simulink model "Systolic_4x4"  (R2021a)
settings: Solver=VariableStepAuto  StartTime=0.0  StopTime=32  RelTol=1e-3
libraries: hdlBasic x195, xbsIndex_r4 x1
(part 1 of 2)
settings Model: Creator=ckk5  LastModifiedBy=ckk5

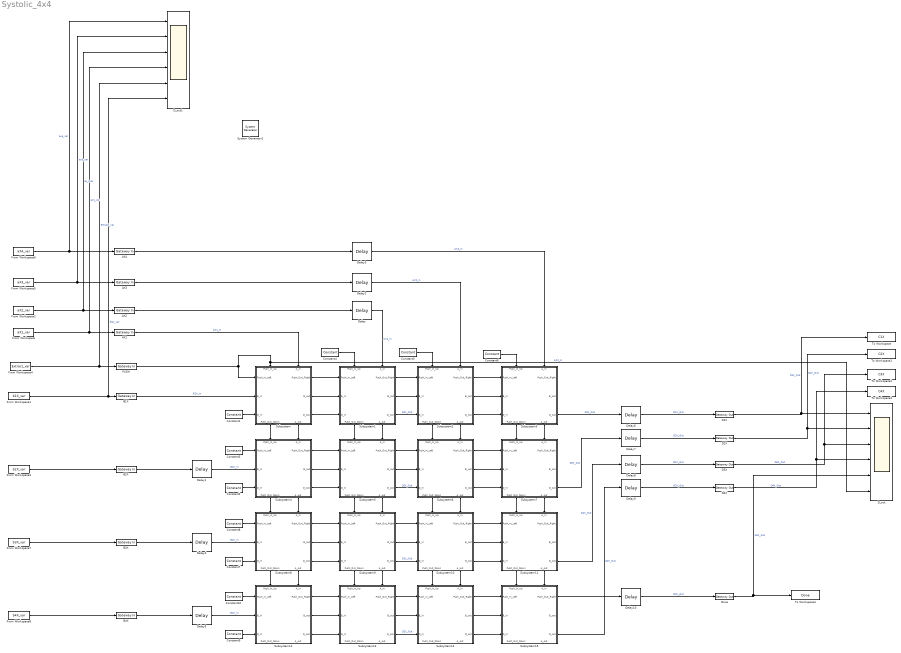
== system Systolic_4x4 ==
  " System Generator1" : xbsIndex_r4/ System Generator  Tag=genX  xilinxfamily=zynq  part=xc7z020  speed=-1  package=clg484  synthesis_tool=Vivado  clock_wrapper=Clock Enables  directory=C:/ELEC522/Cameron/systolic_array_shit  proj_type=Vivado  Synth_file=Vivado Synthesis Defaults  Impl_file=Vivado Implementation Defaults  testbench=off  simulink_period=1  sysclk_period=10  dcm_input_clock_period=10  incr_netlist=off  trim_vbits=Everywhere in SubSystem  dbl_ovrd=According to Block Masks  core_generation=According to Block Masks  run_coregen=off  deprecated_control=off  eval_field=0  block_type=sysgen
  AX{1..4} (4 alike) : hdlBasic/Gateway In  gui_display_data_type=Fixed-point  arith_type=Signed (2's comp)  n_bits=16  bin_pt=0  preci_type=Single  exp_width=8  frac_width=24  rows=1  columns=1  quantization="Round  (unbiased: +/- Inf)"  overflow=Saturate  period=1  UseAsADC=off  ADCChannel='1'  interface=None  automatic_assignment=on  address_offset=hex2dec('00')  intf_name=''  intf_description=''  default_value=0  timing_constraint=None  locs_specified=off  LOCs={}  io_standard={}  inherit_from_input=off  hdl_port=on  XmcBlockStatus=1  maskContainerNames=group4  block_type=gatewayin  block_config=sysgen:gateway_in_config  block_width_w=590  block_height_w=620  block_width=640  block_height=850
  B1X : hdlBasic/Gateway In  gui_display_data_type=Fixed-point  arith_type=Signed (2's comp)  n_bits=16  bin_pt=0  preci_type=Single  exp_width=8  frac_width=24  rows=1  columns=1  quantization="Round  (unbiased: +/- Inf)"  overflow=Saturate  period=1  UseAsADC=off  ADCChannel='1'  interface=None  automatic_assignment=on  address_offset=hex2dec('00')  intf_name=''  intf_description=''  default_value=0  timing_constraint=None  locs_specified=off  LOCs={}  io_standard={}  inherit_from_input=off  hdl_port=on  XmcBlockStatus=1  maskContainerNames=group4  block_type=gatewayin  block_config=sysgen:gateway_in_config  block_width_w=590  block_height_w=620  block_width=640  block_height=850
  B2X : hdlBasic/Gateway In  gui_display_data_type=Fixed-point  arith_type=Signed (2's comp)  n_bits=16  bin_pt=0  preci_type=Single  exp_width=8  frac_width=24  rows=1  columns=1  quantization="Round  (unbiased: +/- Inf)"  overflow=Saturate  period=1  UseAsADC=off  ADCChannel='1'  interface=None  automatic_assignment=on  address_offset=hex2dec('00')  intf_name=''  intf_description=''  default_value=0  timing_constraint=None  locs_specified=off  LOCs={}  io_standard={}  inherit_from_input=off  hdl_port=on  XmcBlockStatus=1  maskContainerNames=group4  block_type=gatewayin  block_config=sysgen:gateway_in_config  block_width_w=590  block_height_w=620  block_width=640  block_height=850
  B3X : hdlBasic/Gateway In  gui_display_data_type=Fixed-point  arith_type=Signed (2's comp)  n_bits=16  bin_pt=0  preci_type=Single  exp_width=8  frac_width=24  rows=1  columns=1  quantization="Round  (unbiased: +/- Inf)"  overflow=Saturate  period=1  UseAsADC=off  ADCChannel='1'  interface=None  automatic_assignment=on  address_offset=hex2dec('00')  intf_name=''  intf_description=''  default_value=0  timing_constraint=None  locs_specified=off  LOCs={}  io_standard={}  inherit_from_input=off  hdl_port=on  XmcBlockStatus=1  maskContainerNames=group4  block_type=gatewayin  block_config=sysgen:gateway_in_config  block_width_w=590  block_height_w=620  block_width=640  block_height=850
  B4X : hdlBasic/Gateway In  gui_display_data_type=Fixed-point  arith_type=Signed (2's comp)  n_bits=16  bin_pt=0  preci_type=Single  exp_width=8  frac_width=24  rows=1  columns=1  quantization="Round  (unbiased: +/- Inf)"  overflow=Saturate  period=1  UseAsADC=off  ADCChannel='1'  interface=None  automatic_assignment=on  address_offset=hex2dec('00')  intf_name=''  intf_description=''  default_value=0  timing_constraint=None  locs_specified=off  LOCs={}  io_standard={}  inherit_from_input=off  hdl_port=on  XmcBlockStatus=1  maskContainerNames=group4  block_type=gatewayin  block_config=sysgen:gateway_in_config  block_width_w=590  block_height_w=620  block_width=640  block_height=850
  Constant{1..2,7,9} (4 alike) : hdlBasic/Constant  const=0  gui_display_data_type=Fixed-point  arith_type=Signed (2's comp)  n_bits=16  bin_pt=0  preci_type=Single  exp_width=8  frac_width=24  explicit_period=off  period=1  XmcBlockStatus=1  maskContainerNames=tabcontainer1  block_type=constant  block_config=sysgen:Constant_config
  Constant{3..6,8,10} (6 alike) : hdlBasic/Constant  const=0  gui_display_data_type=Boolean  arith_type=Boolean  n_bits=16  bin_pt=0  preci_type=Single  exp_width=8  frac_width=24  explicit_period=off  period=1  XmcBlockStatus=1  maskContainerNames=tabcontainer1  block_type=constant  block_config=sysgen:Constant_config
  D1X : hdlBasic/Gateway Out  inherit_from_input=off  hdl_port=on  rows=1  columns=1  UseAsDAC=off  DACChannel='1'  interface=None  automatic_assignment=on  address_offset=hex2dec('00')  intf_name=''  intf_description=''  timing_constraint=None  locs_specified=off  LOCs={}  io_standard={}  XmcBlockStatus=1  maskContainerNames=group4  block_type=gatewayout  block_config=sysgen:gateway_out_config  block_width_w=590  block_height_w=620  block_width=620  block_height=750
  D2X : hdlBasic/Gateway Out  inherit_from_input=off  hdl_port=on  rows=1  columns=1  UseAsDAC=off  DACChannel='1'  interface=None  automatic_assignment=on  address_offset=hex2dec('00')  intf_name=''  intf_description=''  timing_constraint=None  locs_specified=off  LOCs={}  io_standard={}  XmcBlockStatus=1  maskContainerNames=group4  block_type=gatewayout  block_config=sysgen:gateway_out_config  block_width_w=590  block_height_w=620  block_width=620  block_height=750
  D3X : hdlBasic/Gateway Out  inherit_from_input=off  hdl_port=on  rows=1  columns=1  UseAsDAC=off  DACChannel='1'  interface=None  automatic_assignment=on  address_offset=hex2dec('00')  intf_name=''  intf_description=''  timing_constraint=None  locs_specified=off  LOCs={}  io_standard={}  XmcBlockStatus=1  maskContainerNames=group4  block_type=gatewayout  block_config=sysgen:gateway_out_config  block_width_w=590  block_height_w=620  block_width=620  block_height=750
  D4X : hdlBasic/Gateway Out  inherit_from_input=off  hdl_port=on  rows=1  columns=1  UseAsDAC=off  DACChannel='1'  interface=None  automatic_assignment=on  address_offset=hex2dec('00')  intf_name=''  intf_description=''  timing_constraint=None  locs_specified=off  LOCs={}  io_standard={}  XmcBlockStatus=1  maskContainerNames=group4  block_type=gatewayout  block_config=sysgen:gateway_out_config  block_width_w=590  block_height_w=620  block_width=620  block_height=750
  D_out : Scope  NumInputPorts=6
  D_out1 : Scope  NumInputPorts=6
  Delay{,1,9..10} (4 alike) : hdlBasic/Delay  rst=off  en=off  latency=1  reg_retiming=off  XmcBlockStatus=1  maskContainerNames=group1  block_type=delay  block_config=sysgen:Delay_config
  Delay2 : hdlBasic/Delay  rst=off  en=off  latency=2  reg_retiming=off  XmcBlockStatus=1  maskContainerNames=group1  block_type=delay  block_config=sysgen:Delay_config
  Delay3 : hdlBasic/Delay  rst=off  en=off  latency=3  reg_retiming=off  XmcBlockStatus=1  maskContainerNames=group1  block_type=delay  block_config=sysgen:Delay_config
  Delay4 : hdlBasic/Delay  rst=off  en=off  latency=2  reg_retiming=off  XmcBlockStatus=1  maskContainerNames=group1  block_type=delay  block_config=sysgen:Delay_config
  Delay5 : hdlBasic/Delay  rst=off  en=off  latency=3  reg_retiming=off  XmcBlockStatus=1  maskContainerNames=group1  block_type=delay  block_config=sysgen:Delay_config
  Delay6 : hdlBasic/Delay  rst=off  en=off  latency=4  reg_retiming=off  XmcBlockStatus=1  maskContainerNames=group1  block_type=delay  block_config=sysgen:Delay_config
  Delay7 : hdlBasic/Delay  rst=off  en=off  latency=3  reg_retiming=off  XmcBlockStatus=1  maskContainerNames=group1  block_type=delay  block_config=sysgen:Delay_config
  Delay8 : hdlBasic/Delay  rst=off  en=off  latency=2  reg_retiming=off  XmcBlockStatus=1  maskContainerNames=group1  block_type=delay  block_config=sysgen:Delay_config
  Done : hdlBasic/Gateway Out  inherit_from_input=off  hdl_port=on  rows=1  columns=1  UseAsDAC=off  DACChannel='1'  interface=None  automatic_assignment=on  address_offset=hex2dec('00')  intf_name=''  intf_description=''  timing_constraint=None  locs_specified=off  LOCs={}  io_standard={}  XmcBlockStatus=1  maskContainerNames=group4  block_type=gatewayout  block_config=sysgen:gateway_out_config  block_width_w=590  block_height_w=620  block_width=620  block_height=750
  From Workspace : FromWorkspace  VariableName=aX1_var  Interpolate=off  OutputAfterFinalValue=Setting to zero
  From Workspace1 : FromWorkspace  VariableName=b1X_var  Interpolate=off  OutputAfterFinalValue=Setting to zero
  From Workspace2 : FromWorkspace  VariableName=aX2_var  Interpolate=off  OutputAfterFinalValue=Setting to zero
  From Workspace3 : FromWorkspace  VariableName=b2X_var  Interpolate=off  OutputAfterFinalValue=Setting to zero
  From Workspace4 : FromWorkspace  VariableName=Extract_var  Interpolate=off  OutputAfterFinalValue=Setting to zero
  From Workspace5 : FromWorkspace  VariableName=aX3_var  Interpolate=off  OutputAfterFinalValue=Setting to zero
  From Workspace6 : FromWorkspace  VariableName=aX4_var  Interpolate=off  OutputAfterFinalValue=Setting to zero
  From Workspace7 : FromWorkspace  VariableName=b3X_var  Interpolate=off  OutputAfterFinalValue=Setting to zero
  From Workspace8 : FromWorkspace  VariableName=b4X_var  Interpolate=off  OutputAfterFinalValue=Setting to zero
  PUSH : hdlBasic/Gateway In  gui_display_data_type=Boolean  arith_type=Boolean  n_bits=1  bin_pt=0  preci_type=Single  exp_width=8  frac_width=24  rows=1  columns=1  quantization="Round  (unbiased: +/- Inf)"  overflow=Saturate  period=1  UseAsADC=off  ADCChannel='1'  interface=None  automatic_assignment=on  address_offset=hex2dec('00')  intf_name=''  intf_description=''  default_value=0  timing_constraint=None  locs_specified=off  LOCs={}  io_standard={}  inherit_from_input=off  hdl_port=on  XmcBlockStatus=1  maskContainerNames=group4  block_type=gatewayin  block_config=sysgen:gateway_in_config  block_width_w=590  block_height_w=620  block_width=640  block_height=850
  Subsystem : Subsystem
      settings: PortSchema="{\"entries\":[{\"content\":{\"sides\":[{\"content\":{\"connectorIds\":[\"In1\",\"In2\",\"In3\"]},\"type\":\"ConnectorPlacement.EquallySpacedRectSide\",\"uuid\":\"8ff87642-4ab4-4993-8c2d-3e2a0b442edb\"},{\"content\":{\"connectorIds\":[\"Out1\",\"Out2\",\"Out3\"],\"side\":\"RIGHT\"},\"type\":\"ConnectorPlacement.EquallySpacedRectSide\",\"uuid\":\"3e5e616f-4833-4873-80b3-d7c022d50595\"},{\"content\":{\"connectorIds\":[\"In4\",\"In5\"],\"side\":\"TOP\"},\"type\":\"ConnectorPlacement.EquallySpacedRectSide\",\"uuid\":\"e9723aa0-a983-4533-a9ef-daafc8525bc8\"},{\"content\":{\"connectorIds\":[\"Out4\",\"Out5\"],\"side\":\"BOTTOM\"},\"type\":\"ConnectorPlacement.EquallySpacedRectSide\",\"uuid\":\"893be137-9383-4d88-a8a8-bff1bf557b52\"}]},\"type\":\"ConnectorPlacement.EquallySpacedConnector\",\"uuid\":\"84d6313b-76ca-421f-b981-b36aad77f192\"}],\"packageUris\":[\"http://schema.mathworks.com/mf0/Connector/R2020b\"],\"version\":\"1.0\"}"
  Subsystem1 : Subsystem
      settings: PortSchema="{\"entries\":[{\"content\":{\"sides\":[{\"content\":{\"connectorIds\":[\"In1\",\"In2\",\"In3\"]},\"type\":\"ConnectorPlacement.EquallySpacedRectSide\",\"uuid\":\"8ff87642-4ab4-4993-8c2d-3e2a0b442edb\"},{\"content\":{\"connectorIds\":[\"Out1\",\"Out2\",\"Out3\"],\"side\":\"RIGHT\"},\"type\":\"ConnectorPlacement.EquallySpacedRectSide\",\"uuid\":\"3e5e616f-4833-4873-80b3-d7c022d50595\"},{\"content\":{\"connectorIds\":[\"In4\",\"In5\"],\"side\":\"TOP\"},\"type\":\"ConnectorPlacement.EquallySpacedRectSide\",\"uuid\":\"e9723aa0-a983-4533-a9ef-daafc8525bc8\"},{\"content\":{\"connectorIds\":[\"Out4\",\"Out5\"],\"side\":\"BOTTOM\"},\"type\":\"ConnectorPlacement.EquallySpacedRectSide\",\"uuid\":\"893be137-9383-4d88-a8a8-bff1bf557b52\"}]},\"type\":\"ConnectorPlacement.EquallySpacedConnector\",\"uuid\":\"84d6313b-76ca-421f-b981-b36aad77f192\"}],\"packageUris\":[\"http://schema.mathworks.com/mf0/Connector/R2020b\"],\"version\":\"1.0\"}"
  Subsystem10 : Subsystem
      settings: PortSchema="{\"entries\":[{\"content\":{\"sides\":[{\"content\":{\"connectorIds\":[\"In1\",\"In2\",\"In3\"]},\"type\":\"ConnectorPlacement.EquallySpacedRectSide\",\"uuid\":\"8ff87642-4ab4-4993-8c2d-3e2a0b442edb\"},{\"content\":{\"connectorIds\":[\"Out1\",\"Out2\",\"Out3\"],\"side\":\"RIGHT\"},\"type\":\"ConnectorPlacement.EquallySpacedRectSide\",\"uuid\":\"3e5e616f-4833-4873-80b3-d7c022d50595\"},{\"content\":{\"connectorIds\":[\"In4\",\"In5\"],\"side\":\"TOP\"},\"type\":\"ConnectorPlacement.EquallySpacedRectSide\",\"uuid\":\"e9723aa0-a983-4533-a9ef-daafc8525bc8\"},{\"content\":{\"connectorIds\":[\"Out4\",\"Out5\"],\"side\":\"BOTTOM\"},\"type\":\"ConnectorPlacement.EquallySpacedRectSide\",\"uuid\":\"893be137-9383-4d88-a8a8-bff1bf557b52\"}]},\"type\":\"ConnectorPlacement.EquallySpacedConnector\",\"uuid\":\"84d6313b-76ca-421f-b981-b36aad77f192\"}],\"packageUris\":[\"http://schema.mathworks.com/mf0/Connector/R2020b\"],\"version\":\"1.0\"}"
  Subsystem11 : Subsystem
      settings: PortSchema="{\"entries\":[{\"content\":{\"sides\":[{\"content\":{\"connectorIds\":[\"In1\",\"In2\",\"In3\"]},\"type\":\"ConnectorPlacement.EquallySpacedRectSide\",\"uuid\":\"8ff87642-4ab4-4993-8c2d-3e2a0b442edb\"},{\"content\":{\"connectorIds\":[\"Out1\",\"Out2\",\"Out3\"],\"side\":\"RIGHT\"},\"type\":\"ConnectorPlacement.EquallySpacedRectSide\",\"uuid\":\"3e5e616f-4833-4873-80b3-d7c022d50595\"},{\"content\":{\"connectorIds\":[\"In4\",\"In5\"],\"side\":\"TOP\"},\"type\":\"ConnectorPlacement.EquallySpacedRectSide\",\"uuid\":\"e9723aa0-a983-4533-a9ef-daafc8525bc8\"},{\"content\":{\"connectorIds\":[\"Out4\",\"Out5\"],\"side\":\"BOTTOM\"},\"type\":\"ConnectorPlacement.EquallySpacedRectSide\",\"uuid\":\"893be137-9383-4d88-a8a8-bff1bf557b52\"}]},\"type\":\"ConnectorPlacement.EquallySpacedConnector\",\"uuid\":\"84d6313b-76ca-421f-b981-b36aad77f192\"}],\"packageUris\":[\"http://schema.mathworks.com/mf0/Connector/R2020b\"],\"version\":\"1.0\"}"
  Subsystem12 : Subsystem
      settings: PortSchema="{\"entries\":[{\"content\":{\"sides\":[{\"content\":{\"connectorIds\":[\"In1\",\"In2\",\"In3\"]},\"type\":\"ConnectorPlacement.EquallySpacedRectSide\",\"uuid\":\"8ff87642-4ab4-4993-8c2d-3e2a0b442edb\"},{\"content\":{\"connectorIds\":[\"Out1\",\"Out2\",\"Out3\"],\"side\":\"RIGHT\"},\"type\":\"ConnectorPlacement.EquallySpacedRectSide\",\"uuid\":\"3e5e616f-4833-4873-80b3-d7c022d50595\"},{\"content\":{\"connectorIds\":[\"In4\",\"In5\"],\"side\":\"TOP\"},\"type\":\"ConnectorPlacement.EquallySpacedRectSide\",\"uuid\":\"e9723aa0-a983-4533-a9ef-daafc8525bc8\"},{\"content\":{\"connectorIds\":[\"Out4\",\"Out5\"],\"side\":\"BOTTOM\"},\"type\":\"ConnectorPlacement.EquallySpacedRectSide\",\"uuid\":\"893be137-9383-4d88-a8a8-bff1bf557b52\"}]},\"type\":\"ConnectorPlacement.EquallySpacedConnector\",\"uuid\":\"84d6313b-76ca-421f-b981-b36aad77f192\"}],\"packageUris\":[\"http://schema.mathworks.com/mf0/Connector/R2020b\"],\"version\":\"1.0\"}"
  Subsystem13 : Subsystem
      settings: PortSchema="{\"entries\":[{\"content\":{\"sides\":[{\"content\":{\"connectorIds\":[\"In1\",\"In2\",\"In3\"]},\"type\":\"ConnectorPlacement.EquallySpacedRectSide\",\"uuid\":\"8ff87642-4ab4-4993-8c2d-3e2a0b442edb\"},{\"content\":{\"connectorIds\":[\"Out1\",\"Out2\",\"Out3\"],\"side\":\"RIGHT\"},\"type\":\"ConnectorPlacement.EquallySpacedRectSide\",\"uuid\":\"3e5e616f-4833-4873-80b3-d7c022d50595\"},{\"content\":{\"connectorIds\":[\"In4\",\"In5\"],\"side\":\"TOP\"},\"type\":\"ConnectorPlacement.EquallySpacedRectSide\",\"uuid\":\"e9723aa0-a983-4533-a9ef-daafc8525bc8\"},{\"content\":{\"connectorIds\":[\"Out4\",\"Out5\"],\"side\":\"BOTTOM\"},\"type\":\"ConnectorPlacement.EquallySpacedRectSide\",\"uuid\":\"893be137-9383-4d88-a8a8-bff1bf557b52\"}]},\"type\":\"ConnectorPlacement.EquallySpacedConnector\",\"uuid\":\"84d6313b-76ca-421f-b981-b36aad77f192\"}],\"packageUris\":[\"http://schema.mathworks.com/mf0/Connector/R2020b\"],\"version\":\"1.0\"}"
  Subsystem14 : Subsystem
      settings: PortSchema="{\"entries\":[{\"content\":{\"sides\":[{\"content\":{\"connectorIds\":[\"In1\",\"In2\",\"In3\"]},\"type\":\"ConnectorPlacement.EquallySpacedRectSide\",\"uuid\":\"8ff87642-4ab4-4993-8c2d-3e2a0b442edb\"},{\"content\":{\"connectorIds\":[\"Out1\",\"Out2\",\"Out3\"],\"side\":\"RIGHT\"},\"type\":\"ConnectorPlacement.EquallySpacedRectSide\",\"uuid\":\"3e5e616f-4833-4873-80b3-d7c022d50595\"},{\"content\":{\"connectorIds\":[\"In4\",\"In5\"],\"side\":\"TOP\"},\"type\":\"ConnectorPlacement.EquallySpacedRectSide\",\"uuid\":\"e9723aa0-a983-4533-a9ef-daafc8525bc8\"},{\"content\":{\"connectorIds\":[\"Out4\",\"Out5\"],\"side\":\"BOTTOM\"},\"type\":\"ConnectorPlacement.EquallySpacedRectSide\",\"uuid\":\"893be137-9383-4d88-a8a8-bff1bf557b52\"}]},\"type\":\"ConnectorPlacement.EquallySpacedConnector\",\"uuid\":\"84d6313b-76ca-421f-b981-b36aad77f192\"}],\"packageUris\":[\"http://schema.mathworks.com/mf0/Connector/R2020b\"],\"version\":\"1.0\"}"
  Subsystem15 : Subsystem
      settings: PortSchema="{\"entries\":[{\"content\":{\"sides\":[{\"content\":{\"connectorIds\":[\"In1\",\"In2\",\"In3\"]},\"type\":\"ConnectorPlacement.EquallySpacedRectSide\",\"uuid\":\"8ff87642-4ab4-4993-8c2d-3e2a0b442edb\"},{\"content\":{\"connectorIds\":[\"Out1\",\"Out2\",\"Out3\"],\"side\":\"RIGHT\"},\"type\":\"ConnectorPlacement.EquallySpacedRectSide\",\"uuid\":\"3e5e616f-4833-4873-80b3-d7c022d50595\"},{\"content\":{\"connectorIds\":[\"In4\",\"In5\"],\"side\":\"TOP\"},\"type\":\"ConnectorPlacement.EquallySpacedRectSide\",\"uuid\":\"e9723aa0-a983-4533-a9ef-daafc8525bc8\"},{\"content\":{\"connectorIds\":[\"Out4\",\"Out5\"],\"side\":\"BOTTOM\"},\"type\":\"ConnectorPlacement.EquallySpacedRectSide\",\"uuid\":\"893be137-9383-4d88-a8a8-bff1bf557b52\"}]},\"type\":\"ConnectorPlacement.EquallySpacedConnector\",\"uuid\":\"84d6313b-76ca-421f-b981-b36aad77f192\"}],\"packageUris\":[\"http://schema.mathworks.com/mf0/Connector/R2020b\"],\"version\":\"1.0\"}"
  Subsystem2 : Subsystem
      settings: PortSchema="{\"entries\":[{\"content\":{\"sides\":[{\"content\":{\"connectorIds\":[\"In1\",\"In2\",\"In3\"]},\"type\":\"ConnectorPlacement.EquallySpacedRectSide\",\"uuid\":\"8ff87642-4ab4-4993-8c2d-3e2a0b442edb\"},{\"content\":{\"connectorIds\":[\"Out1\",\"Out2\",\"Out3\"],\"side\":\"RIGHT\"},\"type\":\"ConnectorPlacement.EquallySpacedRectSide\",\"uuid\":\"3e5e616f-4833-4873-80b3-d7c022d50595\"},{\"content\":{\"connectorIds\":[\"In4\",\"In5\"],\"side\":\"TOP\"},\"type\":\"ConnectorPlacement.EquallySpacedRectSide\",\"uuid\":\"e9723aa0-a983-4533-a9ef-daafc8525bc8\"},{\"content\":{\"connectorIds\":[\"Out4\",\"Out5\"],\"side\":\"BOTTOM\"},\"type\":\"ConnectorPlacement.EquallySpacedRectSide\",\"uuid\":\"893be137-9383-4d88-a8a8-bff1bf557b52\"}]},\"type\":\"ConnectorPlacement.EquallySpacedConnector\",\"uuid\":\"84d6313b-76ca-421f-b981-b36aad77f192\"}],\"packageUris\":[\"http://schema.mathworks.com/mf0/Connector/R2020b\"],\"version\":\"1.0\"}"
  Subsystem3 : Subsystem
      settings: PortSchema="{\"entries\":[{\"content\":{\"sides\":[{\"content\":{\"connectorIds\":[\"In1\",\"In2\",\"In3\"]},\"type\":\"ConnectorPlacement.EquallySpacedRectSide\",\"uuid\":\"8ff87642-4ab4-4993-8c2d-3e2a0b442edb\"},{\"content\":{\"connectorIds\":[\"Out1\",\"Out2\",\"Out3\"],\"side\":\"RIGHT\"},\"type\":\"ConnectorPlacement.EquallySpacedRectSide\",\"uuid\":\"3e5e616f-4833-4873-80b3-d7c022d50595\"},{\"content\":{\"connectorIds\":[\"In4\",\"In5\"],\"side\":\"TOP\"},\"type\":\"ConnectorPlacement.EquallySpacedRectSide\",\"uuid\":\"e9723aa0-a983-4533-a9ef-daafc8525bc8\"},{\"content\":{\"connectorIds\":[\"Out4\",\"Out5\"],\"side\":\"BOTTOM\"},\"type\":\"ConnectorPlacement.EquallySpacedRectSide\",\"uuid\":\"893be137-9383-4d88-a8a8-bff1bf557b52\"}]},\"type\":\"ConnectorPlacement.EquallySpacedConnector\",\"uuid\":\"84d6313b-76ca-421f-b981-b36aad77f192\"}],\"packageUris\":[\"http://schema.mathworks.com/mf0/Connector/R2020b\"],\"version\":\"1.0\"}"
  Subsystem4 : Subsystem
      settings: PortSchema="{\"entries\":[{\"content\":{\"sides\":[{\"content\":{\"connectorIds\":[\"In1\",\"In2\",\"In3\"]},\"type\":\"ConnectorPlacement.EquallySpacedRectSide\",\"uuid\":\"8ff87642-4ab4-4993-8c2d-3e2a0b442edb\"},{\"content\":{\"connectorIds\":[\"Out1\",\"Out2\",\"Out3\"],\"side\":\"RIGHT\"},\"type\":\"ConnectorPlacement.EquallySpacedRectSide\",\"uuid\":\"3e5e616f-4833-4873-80b3-d7c022d50595\"},{\"content\":{\"connectorIds\":[\"In4\",\"In5\"],\"side\":\"TOP\"},\"type\":\"ConnectorPlacement.EquallySpacedRectSide\",\"uuid\":\"e9723aa0-a983-4533-a9ef-daafc8525bc8\"},{\"content\":{\"connectorIds\":[\"Out4\",\"Out5\"],\"side\":\"BOTTOM\"},\"type\":\"ConnectorPlacement.EquallySpacedRectSide\",\"uuid\":\"893be137-9383-4d88-a8a8-bff1bf557b52\"}]},\"type\":\"ConnectorPlacement.EquallySpacedConnector\",\"uuid\":\"84d6313b-76ca-421f-b981-b36aad77f192\"}],\"packageUris\":[\"http://schema.mathworks.com/mf0/Connector/R2020b\"],\"version\":\"1.0\"}"
  Subsystem5 : Subsystem
      settings: PortSchema="{\"entries\":[{\"content\":{\"sides\":[{\"content\":{\"connectorIds\":[\"In1\",\"In2\",\"In3\"]},\"type\":\"ConnectorPlacement.EquallySpacedRectSide\",\"uuid\":\"8ff87642-4ab4-4993-8c2d-3e2a0b442edb\"},{\"content\":{\"connectorIds\":[\"Out1\",\"Out2\",\"Out3\"],\"side\":\"RIGHT\"},\"type\":\"ConnectorPlacement.EquallySpacedRectSide\",\"uuid\":\"3e5e616f-4833-4873-80b3-d7c022d50595\"},{\"content\":{\"connectorIds\":[\"In4\",\"In5\"],\"side\":\"TOP\"},\"type\":\"ConnectorPlacement.EquallySpacedRectSide\",\"uuid\":\"e9723aa0-a983-4533-a9ef-daafc8525bc8\"},{\"content\":{\"connectorIds\":[\"Out4\",\"Out5\"],\"side\":\"BOTTOM\"},\"type\":\"ConnectorPlacement.EquallySpacedRectSide\",\"uuid\":\"893be137-9383-4d88-a8a8-bff1bf557b52\"}]},\"type\":\"ConnectorPlacement.EquallySpacedConnector\",\"uuid\":\"84d6313b-76ca-421f-b981-b36aad77f192\"}],\"packageUris\":[\"http://schema.mathworks.com/mf0/Connector/R2020b\"],\"version\":\"1.0\"}"
  Subsystem6 : Subsystem
      settings: PortSchema="{\"entries\":[{\"content\":{\"sides\":[{\"content\":{\"connectorIds\":[\"In1\",\"In2\",\"In3\"]},\"type\":\"ConnectorPlacement.EquallySpacedRectSide\",\"uuid\":\"8ff87642-4ab4-4993-8c2d-3e2a0b442edb\"},{\"content\":{\"connectorIds\":[\"Out1\",\"Out2\",\"Out3\"],\"side\":\"RIGHT\"},\"type\":\"ConnectorPlacement.EquallySpacedRectSide\",\"uuid\":\"3e5e616f-4833-4873-80b3-d7c022d50595\"},{\"content\":{\"connectorIds\":[\"In4\",\"In5\"],\"side\":\"TOP\"},\"type\":\"ConnectorPlacement.EquallySpacedRectSide\",\"uuid\":\"e9723aa0-a983-4533-a9ef-daafc8525bc8\"},{\"content\":{\"connectorIds\":[\"Out4\",\"Out5\"],\"side\":\"BOTTOM\"},\"type\":\"ConnectorPlacement.EquallySpacedRectSide\",\"uuid\":\"893be137-9383-4d88-a8a8-bff1bf557b52\"}]},\"type\":\"ConnectorPlacement.EquallySpacedConnector\",\"uuid\":\"84d6313b-76ca-421f-b981-b36aad77f192\"}],\"packageUris\":[\"http://schema.mathworks.com/mf0/Connector/R2020b\"],\"version\":\"1.0\"}"
  Subsystem7 : Subsystem
      settings: PortSchema="{\"entries\":[{\"content\":{\"sides\":[{\"content\":{\"connectorIds\":[\"In1\",\"In2\",\"In3\"]},\"type\":\"ConnectorPlacement.EquallySpacedRectSide\",\"uuid\":\"8ff87642-4ab4-4993-8c2d-3e2a0b442edb\"},{\"content\":{\"connectorIds\":[\"Out1\",\"Out2\",\"Out3\"],\"side\":\"RIGHT\"},\"type\":\"ConnectorPlacement.EquallySpacedRectSide\",\"uuid\":\"3e5e616f-4833-4873-80b3-d7c022d50595\"},{\"content\":{\"connectorIds\":[\"In4\",\"In5\"],\"side\":\"TOP\"},\"type\":\"ConnectorPlacement.EquallySpacedRectSide\",\"uuid\":\"e9723aa0-a983-4533-a9ef-daafc8525bc8\"},{\"content\":{\"connectorIds\":[\"Out4\",\"Out5\"],\"side\":\"BOTTOM\"},\"type\":\"ConnectorPlacement.EquallySpacedRectSide\",\"uuid\":\"893be137-9383-4d88-a8a8-bff1bf557b52\"}]},\"type\":\"ConnectorPlacement.EquallySpacedConnector\",\"uuid\":\"84d6313b-76ca-421f-b981-b36aad77f192\"}],\"packageUris\":[\"http://schema.mathworks.com/mf0/Connector/R2020b\"],\"version\":\"1.0\"}"
  Subsystem8 : Subsystem
      settings: PortSchema="{\"entries\":[{\"content\":{\"sides\":[{\"content\":{\"connectorIds\":[\"In1\",\"In2\",\"In3\"]},\"type\":\"ConnectorPlacement.EquallySpacedRectSide\",\"uuid\":\"8ff87642-4ab4-4993-8c2d-3e2a0b442edb\"},{\"content\":{\"connectorIds\":[\"Out1\",\"Out2\",\"Out3\"],\"side\":\"RIGHT\"},\"type\":\"ConnectorPlacement.EquallySpacedRectSide\",\"uuid\":\"3e5e616f-4833-4873-80b3-d7c022d50595\"},{\"content\":{\"connectorIds\":[\"In4\",\"In5\"],\"side\":\"TOP\"},\"type\":\"ConnectorPlacement.EquallySpacedRectSide\",\"uuid\":\"e9723aa0-a983-4533-a9ef-daafc8525bc8\"},{\"content\":{\"connectorIds\":[\"Out4\",\"Out5\"],\"side\":\"BOTTOM\"},\"type\":\"ConnectorPlacement.EquallySpacedRectSide\",\"uuid\":\"893be137-9383-4d88-a8a8-bff1bf557b52\"}]},\"type\":\"ConnectorPlacement.EquallySpacedConnector\",\"uuid\":\"84d6313b-76ca-421f-b981-b36aad77f192\"}],\"packageUris\":[\"http://schema.mathworks.com/mf0/Connector/R2020b\"],\"version\":\"1.0\"}"
  Subsystem9 : Subsystem
      settings: PortSchema="{\"entries\":[{\"content\":{\"sides\":[{\"content\":{\"connectorIds\":[\"In1\",\"In2\",\"In3\"]},\"type\":\"ConnectorPlacement.EquallySpacedRectSide\",\"uuid\":\"8ff87642-4ab4-4993-8c2d-3e2a0b442edb\"},{\"content\":{\"connectorIds\":[\"Out1\",\"Out2\",\"Out3\"],\"side\":\"RIGHT\"},\"type\":\"ConnectorPlacement.EquallySpacedRectSide\",\"uuid\":\"3e5e616f-4833-4873-80b3-d7c022d50595\"},{\"content\":{\"connectorIds\":[\"In4\",\"In5\"],\"side\":\"TOP\"},\"type\":\"ConnectorPlacement.EquallySpacedRectSide\",\"uuid\":\"e9723aa0-a983-4533-a9ef-daafc8525bc8\"},{\"content\":{\"connectorIds\":[\"Out4\",\"Out5\"],\"side\":\"BOTTOM\"},\"type\":\"ConnectorPlacement.EquallySpacedRectSide\",\"uuid\":\"893be137-9383-4d88-a8a8-bff1bf557b52\"}]},\"type\":\"ConnectorPlacement.EquallySpacedConnector\",\"uuid\":\"84d6313b-76ca-421f-b981-b36aad77f192\"}],\"packageUris\":[\"http://schema.mathworks.com/mf0/Connector/R2020b\"],\"version\":\"1.0\"}"
  To Workspace : ToWorkspace  VariableName=C1X  SaveFormat=Timeseries  SampleTime=-1
  To Workspace1 : ToWorkspace  VariableName=C2X  SaveFormat=Timeseries  SampleTime=-1
  To Workspace2 : ToWorkspace  VariableName=C3X  SaveFormat=Timeseries  SampleTime=-1
  To Workspace3 : ToWorkspace  VariableName=C4X  SaveFormat=Timeseries  SampleTime=-1
  To Workspace4 : ToWorkspace  VariableName=Done  SaveFormat=Timeseries  SampleTime=-1
  wires:
  From Workspace/1 -> D_out1/4, AX1/1  "ax1_var"
  AX1/1 -> Subsystem/5(A_in)  "AX1_In"
  From Workspace1/1 -> D_out1/6, B1X/1  "B1x_var"
  B1X/1 -> Subsystem/2(B_in)  "B1X_In"
  Subsystem1/5(A_out) -> Subsystem5/5(A_in)
  Subsystem1/4(Push_Out_Down) -> Subsystem5/4(Push_In_Up)
  Subsystem/5(A_out) -> Subsystem4/5(A_in)
  Subsystem/4(Push_Out_Down) -> Subsystem4/4(Push_In_Up)
  From Workspace2/1 -> D_out1/3, AX2/1  "ax_2var"
  AX2/1 -> Delay/1
  From Workspace3/1 -> B2X/1
  B2X/1 -> Delay1/1
  Delay/1 -> Subsystem1/5(A_in)  "AX2_In"
  Delay1/1 -> Subsystem4/2(B_in)  "B2X_In"
  From Workspace4/1 -> D_out1/5, PUSH/1  "extract_var"
  Subsystem/1(Push_Out_Right) -> Subsystem1/1(Push_In_Left)
  Subsystem/3(D_out) -> Subsystem1/3(D_in)
  Subsystem4/1(Push_Out_Right) -> Subsystem5/1(Push_In_Left)
  Subsystem4/2(B_out) -> Subsystem5/2(B_in)
  Subsystem4/3(D_out) -> Subsystem5/3(D_in)
  Subsystem/2(B_out) -> Subsystem1/2(B_in)
  Constant2/1 -> Subsystem4/3(D_in)
  Constant3/1 -> Subsystem4/1(Push_In_Left)
  Constant4/1 -> Subsystem1/4(Push_In_Up)
  Subsystem3/3(D_out) -> Delay6/1  "D1X_Out"
  D1X/1 -> To Workspace/1, D_out/1  "D1X_Out"
  Delay7/1 -> D2X/1  "D2X_Out"
  Delay6/1 -> D1X/1  "D1X_Out"
  D2X/1 -> To Workspace1/1, D_out/2  "D2X_Out"
  Subsystem7/3(D_out) -> Delay7/1  "D2X_Out"
  Subsystem2/2(B_out) -> Subsystem3/2(B_in)
  Subsystem2/3(D_out) -> Subsystem3/3(D_in)
  Subsystem6/3(D_out) -> Subsystem7/3(D_in)
  Subsystem3/4(Push_Out_Down) -> Subsystem7/4(Push_In_Up)
  Subsystem2/1(Push_Out_Right) -> Subsystem3/1(Push_In_Left)
  Subsystem6/1(Push_Out_Right) -> Subsystem7/1(Push_In_Left)
  Subsystem3/5(A_out) -> Subsystem7/5(A_in)
  Subsystem6/2(B_out) -> Subsystem7/2(B_in)
  Subsystem2/4(Push_Out_Down) -> Subsystem6/4(Push_In_Up)
  Subsystem2/5(A_out) -> Subsystem6/5(A_in)
  Subsystem8/2(B_out) -> Subsystem9/2(B_in)
  Subsystem8/3(D_out) -> Subsystem9/3(D_in)
  Subsystem12/3(D_out) -> Subsystem13/3(D_in)
  Subsystem9/4(Push_Out_Down) -> Subsystem13/4(Push_In_Up)
  Subsystem8/1(Push_Out_Right) -> Subsystem9/1(Push_In_Left)
  Subsystem12/1(Push_Out_Right) -> Subsystem13/1(Push_In_Left)
  Subsystem9/5(A_out) -> Subsystem13/5(A_in)
  Subsystem12/2(B_out) -> Subsystem13/2(B_in)
  Subsystem8/4(Push_Out_Down) -> Subsystem12/4(Push_In_Up)
  Subsystem8/5(A_out) -> Subsystem12/5(A_in)
  Subsystem5/5(A_out) -> Subsystem9/5(A_in)
  Subsystem5/4(Push_Out_Down) -> Subsystem9/4(Push_In_Up)
  Subsystem10/2(B_out) -> Subsystem11/2(B_in)
  Subsystem10/3(D_out) -> Subsystem11/3(D_in)
  Subsystem14/3(D_out) -> Subsystem15/3(D_in)
  Subsystem11/4(Push_Out_Down) -> Subsystem15/4(Push_In_Up)
  Subsystem10/1(Push_Out_Right) -> Subsystem11/1(Push_In_Left)
  Subsystem14/1(Push_Out_Right) -> Subsystem15/1(Push_In_Left)
  Subsystem11/5(A_out) -> Subsystem15/5(A_in)
  Subsystem14/2(B_out) -> Subsystem15/2(B_in)
  Subsystem7/4(Push_Out_Down) -> Subsystem11/4(Push_In_Up)
  Subsystem7/5(A_out) -> Subsystem11/5(A_in)
  Subsystem6/5(A_out) -> Subsystem10/5(A_in)
  Subsystem6/4(Push_Out_Down) -> Subsystem10/4(Push_In_Up)
  Subsystem9/1(Push_Out_Right) -> Subsystem10/1(Push_In_Left)
  Subsystem9/2(B_out) -> Subsystem10/2(B_in)
  Subsystem9/3(D_out) -> Subsystem10/3(D_in)  "D1X_Out"
  Subsystem13/1(Push_Out_Right) -> Subsystem14/1(Push_In_Left)
  Subsystem13/2(B_out) -> Subsystem14/2(B_in)
  Subsystem13/3(D_out) -> Subsystem14/3(D_in)  "D2X_Out"
  Subsystem5/3(D_out) -> Subsystem6/3(D_in)  "D2X_Out"
  Subsystem5/2(B_out) -> Subsystem6/2(B_in)
  Subsystem5/1(Push_Out_Right) -> Subsystem6/1(Push_In_Left)
  Subsystem1/3(D_out) -> Subsystem2/3(D_in)  "D1X_Out"
  Subsystem1/2(B_out) -> Subsystem2/2(B_in)
  Subsystem1/1(Push_Out_Right) -> Subsystem2/1(Push_In_Left)
  AX3/1 -> Delay2/1
  From Workspace5/1 -> D_out1/2, AX3/1  "ax3_var"
  AX4/1 -> Delay3/1
  From Workspace6/1 -> D_out1/1, AX4/1  "ax4_var"
  Delay2/1 -> Subsystem2/5(A_in)  "AX2_In"
  Delay3/1 -> Subsystem3/5(A_in)  "AX2_In"
  Constant5/1 -> Subsystem2/4(Push_In_Up)
  Constant6/1 -> Subsystem3/4(Push_In_Up)
  Constant8/1 -> Subsystem8/1(Push_In_Left)
  Delay4/1 -> Subsystem8/2(B_in)  "B2X_In"
  B3X/1 -> Delay4/1
  From Workspace7/1 -> B3X/1
  Constant7/1 -> Subsystem8/3(D_in)
  Constant10/1 -> Subsystem12/1(Push_In_Left)
  Delay5/1 -> Subsystem12/2(B_in)  "B2X_In"
  B4X/1 -> Delay5/1
  From Workspace8/1 -> B4X/1
  Constant9/1 -> Subsystem12/3(D_in)
  Subsystem11/3(D_out) -> Delay8/1  "D1X_Out"
  Delay8/1 -> D3X/1  "D1X_Out"
  Delay9/1 -> D4X/1  "D2X_Out"
  Subsystem15/3(D_out) -> Delay9/1  "D2X_Out"
  Subsystem4/4(Push_Out_Down) -> Subsystem8/4(Push_In_Up)
  Subsystem4/5(A_out) -> Subsystem8/5(A_in)
  Subsystem15/1(Push_Out_Right) -> Delay10/1
  D4X/1 -> D_out/4, To Workspace3/1  "D4X_Out"
  D3X/1 -> To Workspace2/1, D_out/3  "D3X_Out"
  Constant1/1 -> Subsystem/3(D_in)
  PUSH/1 -> D_out/6, Subsystem/4(Push_In_Up), Subsystem/1(Push_In_Left)  "AX2_In"
  Subsystem10/5(A_out) -> Subsystem14/5(A_in)
  Subsystem10/4(Push_Out_Down) -> Subsystem14/4(Push_In_Up)
  Done/1 -> To Workspace4/1, D_out/5  "D4X_Out"
  Delay10/1 -> Done/1  "D2X_Out"

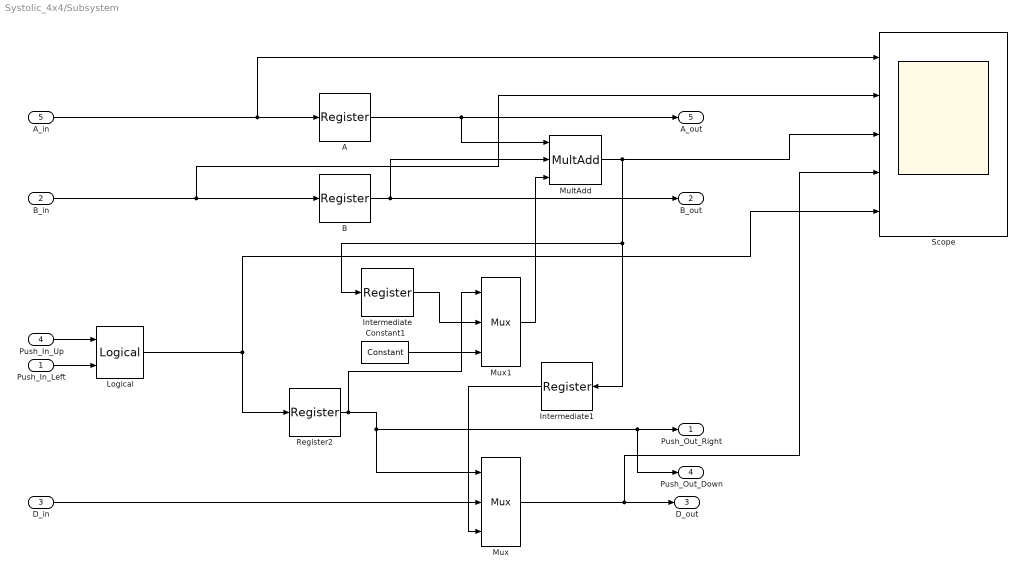
== system Systolic_4x4/Subsystem ==
  Push_In_Left : Inport
  B_in : Inport  Port=2
  D_in : Inport  Port=3
  Push_In_Up : Inport  Port=4
  A_in : Inport  Port=5
  A : hdlBasic/Register  init=0  rst=off  en=off  XmcBlockStatus=1  maskContainerNames=tabcontainer1  block_type=register  block_config=sysgen:Register_config
  B : hdlBasic/Register  init=0  rst=off  en=off  XmcBlockStatus=1  maskContainerNames=tabcontainer1  block_type=register  block_config=sysgen:Register_config
  Constant1 : hdlBasic/Constant  const=0  gui_display_data_type=Fixed-point  arith_type=Signed (2's comp)  n_bits=16  bin_pt=0  preci_type=Single  exp_width=8  frac_width=24  explicit_period=off  period=1  XmcBlockStatus=1  maskContainerNames=tabcontainer1  block_type=constant  block_config=sysgen:Constant_config
  Intermediate : hdlBasic/Register  init=0  rst=off  en=off  XmcBlockStatus=1  maskContainerNames=tabcontainer1  block_type=register  block_config=sysgen:Register_config
  Intermediate1 : hdlBasic/Register  init=0  rst=off  en=off  XmcBlockStatus=1  maskContainerNames=tabcontainer1  block_type=register  block_config=sysgen:Register_config
  Logical : hdlBasic/Logical  logical_function=OR  inputs=2  en=off  latency=0  precision=Full  arith_type=Unsigned  n_bits=16  bin_pt=0  align_bp=on  overflow=[]  quantization=[]  XmcBlockStatus=1  maskContainerNames=tabcontainer1  block_type=logical  block_config=sysgen:Logical_config
  MultAdd : hdlBasic/MultAdd  mode=Addition  en=off  latency=0  precision=Full  arith_type=Unsigned  n_bits=16  bin_pt=14  XmcBlockStatus=1  maskContainerNames=tabcontainer1  block_type=multadd  block_config=sysgen:MultAdd_config
  Mux : hdlBasic/Mux  inputs=2  en=off  latency=0  precision=User Defined  arith_type=Unsigned  n_bits=16  bin_pt=0  quantization=Truncate  overflow=Wrap  XmcBlockStatus=1  maskContainerNames=tabcontainer1  block_type=mux  block_config=sysgen:Mux_config
  Mux1 : hdlBasic/Mux  inputs=2  en=off  latency=0  precision=User Defined  arith_type=Unsigned  n_bits=16  bin_pt=0  quantization=Truncate  overflow=Wrap  XmcBlockStatus=1  maskContainerNames=tabcontainer1  block_type=mux  block_config=sysgen:Mux_config
  Register2 : hdlBasic/Register  init=0  rst=off  en=off  XmcBlockStatus=1  maskContainerNames=tabcontainer1  block_type=register  block_config=sysgen:Register_config
  Scope : Scope  NumInputPorts=5
  Push_Out_Right : Outport
  B_out : Outport  Port=2
  D_out : Outport  Port=3
  Push_Out_Down : Outport  Port=4
  A_out : Outport  Port=5
  wires:
  A/1 -> MultAdd/1, A_out/1
  B/1 -> MultAdd/2, B_out/1
  B_in/1 -> Scope/2, B/1
  A_in/1 -> Scope/1, A/1
  Mux/1 -> Scope/4, D_out/1
  D_in/1 -> Mux/2
  Push_In_Left/1 -> Logical/2
  Push_In_Up/1 -> Logical/1
  Register2/1 -> Mux1/1, Mux/1, Push_Out_Down/1, Push_Out_Right/1
  Logical/1 -> Scope/5, Register2/1
  Intermediate/1 -> Mux1/2
  Mux1/1 -> MultAdd/3
  Constant1/1 -> Mux1/3
  MultAdd/1 -> Scope/3, Intermediate1/1, Intermediate/1
  Intermediate1/1 -> Mux/3

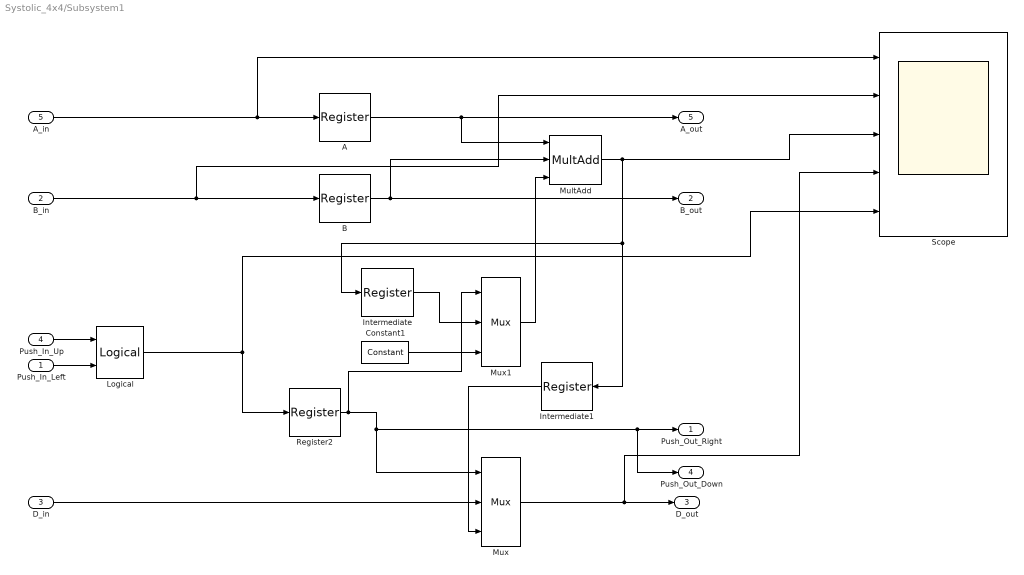
== system Systolic_4x4/Subsystem1 ==
  Push_In_Left : Inport
  B_in : Inport  Port=2
  D_in : Inport  Port=3
  Push_In_Up : Inport  Port=4
  A_in : Inport  Port=5
  A : hdlBasic/Register  init=0  rst=off  en=off  XmcBlockStatus=1  maskContainerNames=tabcontainer1  block_type=register  block_config=sysgen:Register_config
  B : hdlBasic/Register  init=0  rst=off  en=off  XmcBlockStatus=1  maskContainerNames=tabcontainer1  block_type=register  block_config=sysgen:Register_config
  Constant1 : hdlBasic/Constant  const=0  gui_display_data_type=Fixed-point  arith_type=Signed (2's comp)  n_bits=16  bin_pt=0  preci_type=Single  exp_width=8  frac_width=24  explicit_period=off  period=1  XmcBlockStatus=1  maskContainerNames=tabcontainer1  block_type=constant  block_config=sysgen:Constant_config
  Intermediate : hdlBasic/Register  init=0  rst=off  en=off  XmcBlockStatus=1  maskContainerNames=tabcontainer1  block_type=register  block_config=sysgen:Register_config
  Intermediate1 : hdlBasic/Register  init=0  rst=off  en=off  XmcBlockStatus=1  maskContainerNames=tabcontainer1  block_type=register  block_config=sysgen:Register_config
  Logical : hdlBasic/Logical  logical_function=OR  inputs=2  en=off  latency=0  precision=Full  arith_type=Unsigned  n_bits=16  bin_pt=0  align_bp=on  overflow=[]  quantization=[]  XmcBlockStatus=1  maskContainerNames=tabcontainer1  block_type=logical  block_config=sysgen:Logical_config
  MultAdd : hdlBasic/MultAdd  mode=Addition  en=off  latency=0  precision=Full  arith_type=Unsigned  n_bits=16  bin_pt=14  XmcBlockStatus=1  maskContainerNames=tabcontainer1  block_type=multadd  block_config=sysgen:MultAdd_config
  Mux : hdlBasic/Mux  inputs=2  en=off  latency=0  precision=User Defined  arith_type=Unsigned  n_bits=16  bin_pt=0  quantization=Truncate  overflow=Wrap  XmcBlockStatus=1  maskContainerNames=tabcontainer1  block_type=mux  block_config=sysgen:Mux_config
  Mux1 : hdlBasic/Mux  inputs=2  en=off  latency=0  precision=User Defined  arith_type=Unsigned  n_bits=16  bin_pt=0  quantization=Truncate  overflow=Wrap  XmcBlockStatus=1  maskContainerNames=tabcontainer1  block_type=mux  block_config=sysgen:Mux_config
  Register2 : hdlBasic/Register  init=0  rst=off  en=off  XmcBlockStatus=1  maskContainerNames=tabcontainer1  block_type=register  block_config=sysgen:Register_config
  Scope : Scope  NumInputPorts=5
  Push_Out_Right : Outport
  B_out : Outport  Port=2
  D_out : Outport  Port=3
  Push_Out_Down : Outport  Port=4
  A_out : Outport  Port=5
  wires:
  A/1 -> MultAdd/1, A_out/1
  B/1 -> MultAdd/2, B_out/1
  B_in/1 -> Scope/2, B/1
  A_in/1 -> Scope/1, A/1
  Mux/1 -> Scope/4, D_out/1
  D_in/1 -> Mux/2
  Push_In_Left/1 -> Logical/2
  Push_In_Up/1 -> Logical/1
  Register2/1 -> Mux1/1, Mux/1, Push_Out_Down/1, Push_Out_Right/1
  Logical/1 -> Scope/5, Register2/1
  Intermediate/1 -> Mux1/2
  Mux1/1 -> MultAdd/3
  Constant1/1 -> Mux1/3
  MultAdd/1 -> Scope/3, Intermediate1/1, Intermediate/1
  Intermediate1/1 -> Mux/3

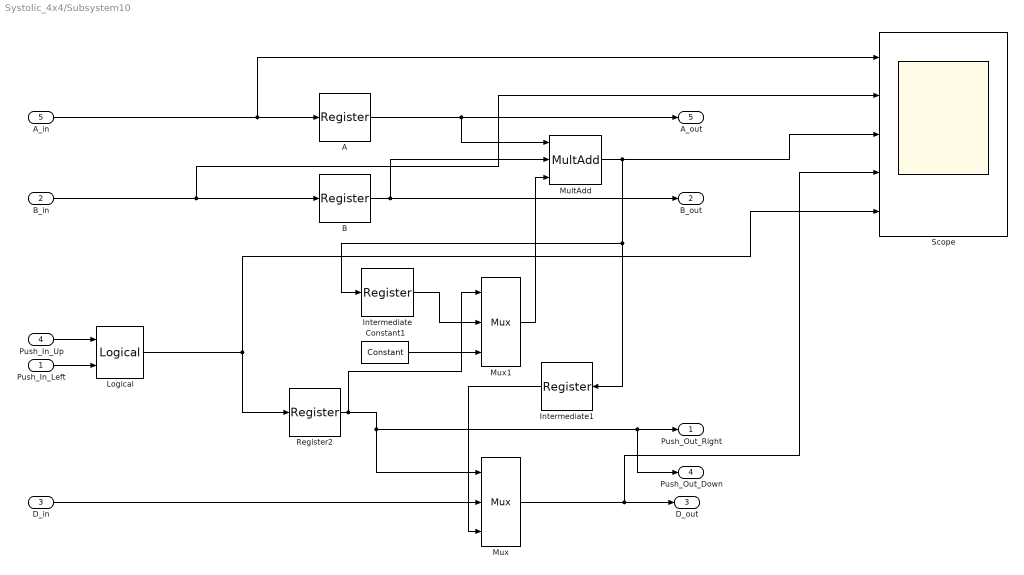
== system Systolic_4x4/Subsystem10 ==
  Push_In_Left : Inport
  B_in : Inport  Port=2
  D_in : Inport  Port=3
  Push_In_Up : Inport  Port=4
  A_in : Inport  Port=5
  A : hdlBasic/Register  init=0  rst=off  en=off  XmcBlockStatus=1  maskContainerNames=tabcontainer1  block_type=register  block_config=sysgen:Register_config
  B : hdlBasic/Register  init=0  rst=off  en=off  XmcBlockStatus=1  maskContainerNames=tabcontainer1  block_type=register  block_config=sysgen:Register_config
  Constant1 : hdlBasic/Constant  const=0  gui_display_data_type=Fixed-point  arith_type=Signed (2's comp)  n_bits=16  bin_pt=0  preci_type=Single  exp_width=8  frac_width=24  explicit_period=off  period=1  XmcBlockStatus=1  maskContainerNames=tabcontainer1  block_type=constant  block_config=sysgen:Constant_config
  Intermediate : hdlBasic/Register  init=0  rst=off  en=off  XmcBlockStatus=1  maskContainerNames=tabcontainer1  block_type=register  block_config=sysgen:Register_config
  Intermediate1 : hdlBasic/Register  init=0  rst=off  en=off  XmcBlockStatus=1  maskContainerNames=tabcontainer1  block_type=register  block_config=sysgen:Register_config
  Logical : hdlBasic/Logical  logical_function=OR  inputs=2  en=off  latency=0  precision=Full  arith_type=Unsigned  n_bits=16  bin_pt=0  align_bp=on  overflow=[]  quantization=[]  XmcBlockStatus=1  maskContainerNames=tabcontainer1  block_type=logical  block_config=sysgen:Logical_config
  MultAdd : hdlBasic/MultAdd  mode=Addition  en=off  latency=0  precision=Full  arith_type=Unsigned  n_bits=16  bin_pt=14  XmcBlockStatus=1  maskContainerNames=tabcontainer1  block_type=multadd  block_config=sysgen:MultAdd_config
  Mux : hdlBasic/Mux  inputs=2  en=off  latency=0  precision=User Defined  arith_type=Unsigned  n_bits=16  bin_pt=0  quantization=Truncate  overflow=Wrap  XmcBlockStatus=1  maskContainerNames=tabcontainer1  block_type=mux  block_config=sysgen:Mux_config
  Mux1 : hdlBasic/Mux  inputs=2  en=off  latency=0  precision=User Defined  arith_type=Unsigned  n_bits=16  bin_pt=0  quantization=Truncate  overflow=Wrap  XmcBlockStatus=1  maskContainerNames=tabcontainer1  block_type=mux  block_config=sysgen:Mux_config
  Register2 : hdlBasic/Register  init=0  rst=off  en=off  XmcBlockStatus=1  maskContainerNames=tabcontainer1  block_type=register  block_config=sysgen:Register_config
  Scope : Scope  NumInputPorts=5
  Push_Out_Right : Outport
  B_out : Outport  Port=2
  D_out : Outport  Port=3
  Push_Out_Down : Outport  Port=4
  A_out : Outport  Port=5
  wires:
  A/1 -> MultAdd/1, A_out/1
  B/1 -> MultAdd/2, B_out/1
  B_in/1 -> Scope/2, B/1
  A_in/1 -> Scope/1, A/1
  Mux/1 -> Scope/4, D_out/1
  D_in/1 -> Mux/2
  Push_In_Left/1 -> Logical/2
  Push_In_Up/1 -> Logical/1
  Register2/1 -> Mux1/1, Mux/1, Push_Out_Down/1, Push_Out_Right/1
  Logical/1 -> Scope/5, Register2/1
  Intermediate/1 -> Mux1/2
  Mux1/1 -> MultAdd/3
  Constant1/1 -> Mux1/3
  MultAdd/1 -> Scope/3, Intermediate1/1, Intermediate/1
  Intermediate1/1 -> Mux/3

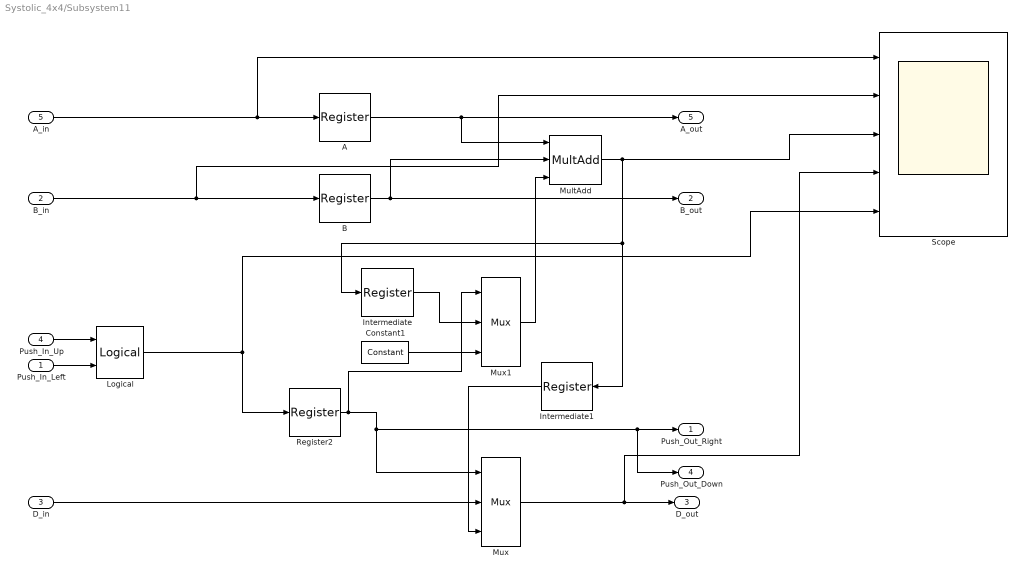
== system Systolic_4x4/Subsystem11 ==
  Push_In_Left : Inport
  B_in : Inport  Port=2
  D_in : Inport  Port=3
  Push_In_Up : Inport  Port=4
  A_in : Inport  Port=5
  A : hdlBasic/Register  init=0  rst=off  en=off  XmcBlockStatus=1  maskContainerNames=tabcontainer1  block_type=register  block_config=sysgen:Register_config
  B : hdlBasic/Register  init=0  rst=off  en=off  XmcBlockStatus=1  maskContainerNames=tabcontainer1  block_type=register  block_config=sysgen:Register_config
  Constant1 : hdlBasic/Constant  const=0  gui_display_data_type=Fixed-point  arith_type=Signed (2's comp)  n_bits=16  bin_pt=0  preci_type=Single  exp_width=8  frac_width=24  explicit_period=off  period=1  XmcBlockStatus=1  maskContainerNames=tabcontainer1  block_type=constant  block_config=sysgen:Constant_config
  Intermediate : hdlBasic/Register  init=0  rst=off  en=off  XmcBlockStatus=1  maskContainerNames=tabcontainer1  block_type=register  block_config=sysgen:Register_config
  Intermediate1 : hdlBasic/Register  init=0  rst=off  en=off  XmcBlockStatus=1  maskContainerNames=tabcontainer1  block_type=register  block_config=sysgen:Register_config
  Logical : hdlBasic/Logical  logical_function=OR  inputs=2  en=off  latency=0  precision=Full  arith_type=Unsigned  n_bits=16  bin_pt=0  align_bp=on  overflow=[]  quantization=[]  XmcBlockStatus=1  maskContainerNames=tabcontainer1  block_type=logical  block_config=sysgen:Logical_config
  MultAdd : hdlBasic/MultAdd  mode=Addition  en=off  latency=0  precision=Full  arith_type=Unsigned  n_bits=16  bin_pt=14  XmcBlockStatus=1  maskContainerNames=tabcontainer1  block_type=multadd  block_config=sysgen:MultAdd_config
  Mux : hdlBasic/Mux  inputs=2  en=off  latency=0  precision=User Defined  arith_type=Unsigned  n_bits=16  bin_pt=0  quantization=Truncate  overflow=Wrap  XmcBlockStatus=1  maskContainerNames=tabcontainer1  block_type=mux  block_config=sysgen:Mux_config
  Mux1 : hdlBasic/Mux  inputs=2  en=off  latency=0  precision=User Defined  arith_type=Unsigned  n_bits=16  bin_pt=0  quantization=Truncate  overflow=Wrap  XmcBlockStatus=1  maskContainerNames=tabcontainer1  block_type=mux  block_config=sysgen:Mux_config
  Register2 : hdlBasic/Register  init=0  rst=off  en=off  XmcBlockStatus=1  maskContainerNames=tabcontainer1  block_type=register  block_config=sysgen:Register_config
  Scope : Scope  NumInputPorts=5
  Push_Out_Right : Outport
  B_out : Outport  Port=2
  D_out : Outport  Port=3
  Push_Out_Down : Outport  Port=4
  A_out : Outport  Port=5
  wires:
  A/1 -> MultAdd/1, A_out/1
  B/1 -> MultAdd/2, B_out/1
  B_in/1 -> Scope/2, B/1
  A_in/1 -> Scope/1, A/1
  Mux/1 -> Scope/4, D_out/1
  D_in/1 -> Mux/2
  Push_In_Left/1 -> Logical/2
  Push_In_Up/1 -> Logical/1
  Register2/1 -> Mux1/1, Mux/1, Push_Out_Down/1, Push_Out_Right/1
  Logical/1 -> Scope/5, Register2/1
  Intermediate/1 -> Mux1/2
  Mux1/1 -> MultAdd/3
  Constant1/1 -> Mux1/3
  MultAdd/1 -> Scope/3, Intermediate1/1, Intermediate/1
  Intermediate1/1 -> Mux/3

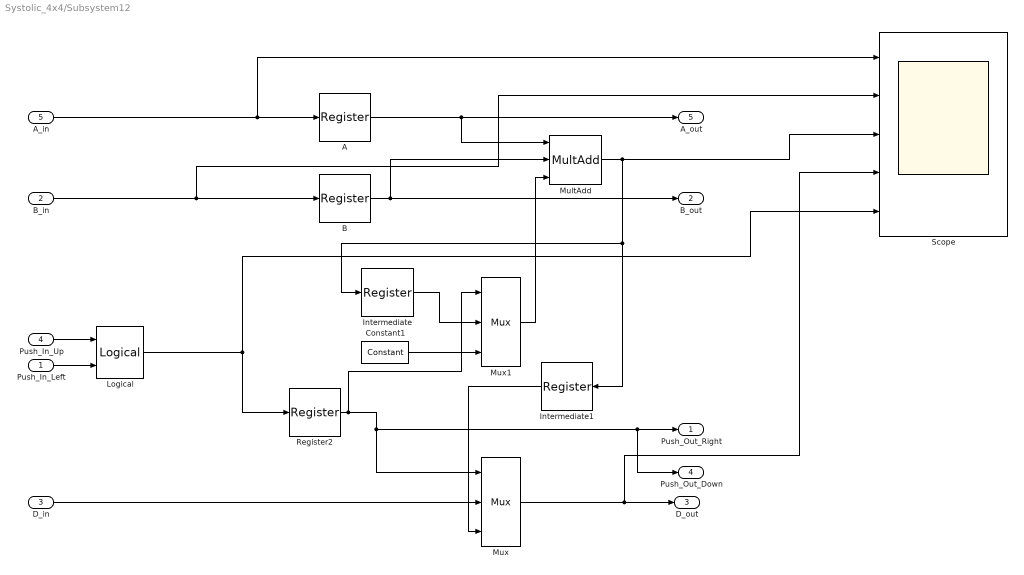
== system Systolic_4x4/Subsystem12 ==
  Push_In_Left : Inport
  B_in : Inport  Port=2
  D_in : Inport  Port=3
  Push_In_Up : Inport  Port=4
  A_in : Inport  Port=5
  A : hdlBasic/Register  init=0  rst=off  en=off  XmcBlockStatus=1  maskContainerNames=tabcontainer1  block_type=register  block_config=sysgen:Register_config
  B : hdlBasic/Register  init=0  rst=off  en=off  XmcBlockStatus=1  maskContainerNames=tabcontainer1  block_type=register  block_config=sysgen:Register_config
  Constant1 : hdlBasic/Constant  const=0  gui_display_data_type=Fixed-point  arith_type=Signed (2's comp)  n_bits=16  bin_pt=0  preci_type=Single  exp_width=8  frac_width=24  explicit_period=off  period=1  XmcBlockStatus=1  maskContainerNames=tabcontainer1  block_type=constant  block_config=sysgen:Constant_config
  Intermediate : hdlBasic/Register  init=0  rst=off  en=off  XmcBlockStatus=1  maskContainerNames=tabcontainer1  block_type=register  block_config=sysgen:Register_config
  Intermediate1 : hdlBasic/Register  init=0  rst=off  en=off  XmcBlockStatus=1  maskContainerNames=tabcontainer1  block_type=register  block_config=sysgen:Register_config
  Logical : hdlBasic/Logical  logical_function=OR  inputs=2  en=off  latency=0  precision=Full  arith_type=Unsigned  n_bits=16  bin_pt=0  align_bp=on  overflow=[]  quantization=[]  XmcBlockStatus=1  maskContainerNames=tabcontainer1  block_type=logical  block_config=sysgen:Logical_config
  MultAdd : hdlBasic/MultAdd  mode=Addition  en=off  latency=0  precision=Full  arith_type=Unsigned  n_bits=16  bin_pt=14  XmcBlockStatus=1  maskContainerNames=tabcontainer1  block_type=multadd  block_config=sysgen:MultAdd_config
  Mux : hdlBasic/Mux  inputs=2  en=off  latency=0  precision=User Defined  arith_type=Unsigned  n_bits=16  bin_pt=0  quantization=Truncate  overflow=Wrap  XmcBlockStatus=1  maskContainerNames=tabcontainer1  block_type=mux  block_config=sysgen:Mux_config
  Mux1 : hdlBasic/Mux  inputs=2  en=off  latency=0  precision=User Defined  arith_type=Unsigned  n_bits=16  bin_pt=0  quantization=Truncate  overflow=Wrap  XmcBlockStatus=1  maskContainerNames=tabcontainer1  block_type=mux  block_config=sysgen:Mux_config
  Register2 : hdlBasic/Register  init=0  rst=off  en=off  XmcBlockStatus=1  maskContainerNames=tabcontainer1  block_type=register  block_config=sysgen:Register_config
  Scope : Scope  NumInputPorts=5
  Push_Out_Right : Outport
  B_out : Outport  Port=2
  D_out : Outport  Port=3
  Push_Out_Down : Outport  Port=4
  A_out : Outport  Port=5
  wires:
  A/1 -> MultAdd/1, A_out/1
  B/1 -> MultAdd/2, B_out/1
  B_in/1 -> Scope/2, B/1
  A_in/1 -> Scope/1, A/1
  Mux/1 -> Scope/4, D_out/1
  D_in/1 -> Mux/2
  Push_In_Left/1 -> Logical/2
  Push_In_Up/1 -> Logical/1
  Register2/1 -> Mux1/1, Mux/1, Push_Out_Down/1, Push_Out_Right/1
  Logical/1 -> Scope/5, Register2/1
  Intermediate/1 -> Mux1/2
  Mux1/1 -> MultAdd/3
  Constant1/1 -> Mux1/3
  MultAdd/1 -> Scope/3, Intermediate1/1, Intermediate/1
  Intermediate1/1 -> Mux/3

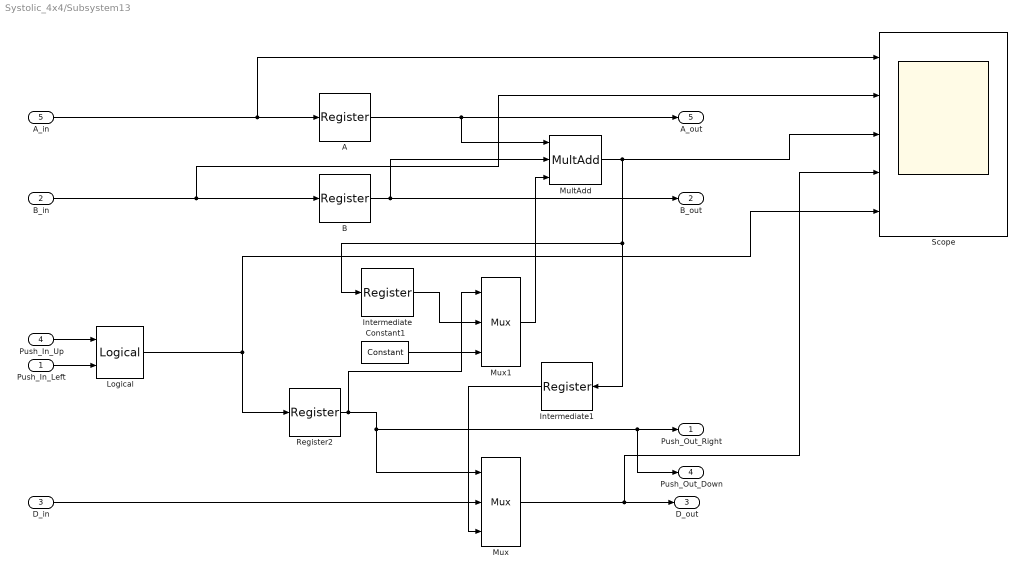
== system Systolic_4x4/Subsystem13 ==
  Push_In_Left : Inport
  B_in : Inport  Port=2
  D_in : Inport  Port=3
  Push_In_Up : Inport  Port=4
  A_in : Inport  Port=5
  A : hdlBasic/Register  init=0  rst=off  en=off  XmcBlockStatus=1  maskContainerNames=tabcontainer1  block_type=register  block_config=sysgen:Register_config
  B : hdlBasic/Register  init=0  rst=off  en=off  XmcBlockStatus=1  maskContainerNames=tabcontainer1  block_type=register  block_config=sysgen:Register_config
  Constant1 : hdlBasic/Constant  const=0  gui_display_data_type=Fixed-point  arith_type=Signed (2's comp)  n_bits=16  bin_pt=0  preci_type=Single  exp_width=8  frac_width=24  explicit_period=off  period=1  XmcBlockStatus=1  maskContainerNames=tabcontainer1  block_type=constant  block_config=sysgen:Constant_config
  Intermediate : hdlBasic/Register  init=0  rst=off  en=off  XmcBlockStatus=1  maskContainerNames=tabcontainer1  block_type=register  block_config=sysgen:Register_config
  Intermediate1 : hdlBasic/Register  init=0  rst=off  en=off  XmcBlockStatus=1  maskContainerNames=tabcontainer1  block_type=register  block_config=sysgen:Register_config
  Logical : hdlBasic/Logical  logical_function=OR  inputs=2  en=off  latency=0  precision=Full  arith_type=Unsigned  n_bits=16  bin_pt=0  align_bp=on  overflow=[]  quantization=[]  XmcBlockStatus=1  maskContainerNames=tabcontainer1  block_type=logical  block_config=sysgen:Logical_config
  MultAdd : hdlBasic/MultAdd  mode=Addition  en=off  latency=0  precision=Full  arith_type=Unsigned  n_bits=16  bin_pt=14  XmcBlockStatus=1  maskContainerNames=tabcontainer1  block_type=multadd  block_config=sysgen:MultAdd_config
  Mux : hdlBasic/Mux  inputs=2  en=off  latency=0  precision=User Defined  arith_type=Unsigned  n_bits=16  bin_pt=0  quantization=Truncate  overflow=Wrap  XmcBlockStatus=1  maskContainerNames=tabcontainer1  block_type=mux  block_config=sysgen:Mux_config
  Mux1 : hdlBasic/Mux  inputs=2  en=off  latency=0  precision=User Defined  arith_type=Unsigned  n_bits=16  bin_pt=0  quantization=Truncate  overflow=Wrap  XmcBlockStatus=1  maskContainerNames=tabcontainer1  block_type=mux  block_config=sysgen:Mux_config
  Register2 : hdlBasic/Register  init=0  rst=off  en=off  XmcBlockStatus=1  maskContainerNames=tabcontainer1  block_type=register  block_config=sysgen:Register_config
  Scope : Scope  NumInputPorts=5
  Push_Out_Right : Outport
  B_out : Outport  Port=2
  D_out : Outport  Port=3
  Push_Out_Down : Outport  Port=4
  A_out : Outport  Port=5
  wires:
  A/1 -> MultAdd/1, A_out/1
  B/1 -> MultAdd/2, B_out/1
  B_in/1 -> Scope/2, B/1
  A_in/1 -> Scope/1, A/1
  Mux/1 -> Scope/4, D_out/1
  D_in/1 -> Mux/2
  Push_In_Left/1 -> Logical/2
  Push_In_Up/1 -> Logical/1
  Register2/1 -> Mux1/1, Mux/1, Push_Out_Down/1, Push_Out_Right/1
  Logical/1 -> Scope/5, Register2/1
  Intermediate/1 -> Mux1/2
  Mux1/1 -> MultAdd/3
  Constant1/1 -> Mux1/3
  MultAdd/1 -> Scope/3, Intermediate1/1, Intermediate/1
  Intermediate1/1 -> Mux/3
